simulink model "trirtyfour"  (R2022b)
settings: Solver=VariableStepAuto  StartTime=0.0  StopTime=10.0  RelTol=1e-3
settings Model: Creator=User  LastModifiedBy=User

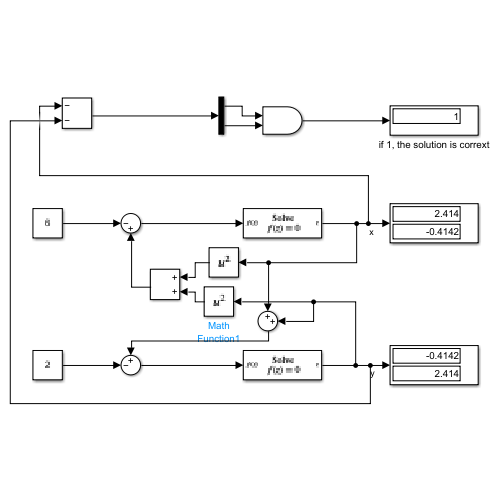
[thumbnail: Simulink's stored preview of the top-level diagram]
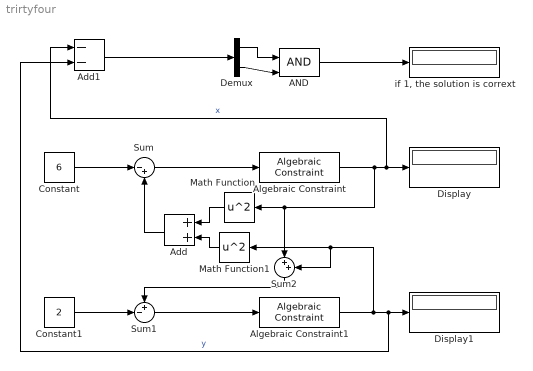
== system trirtyfour ==
  AND : Logic  IconShape=distinctive  AllPortsSameDT=off  OutDataTypeStr=boolean
  Add : Sum
  Add1 : Sum  Inputs=--
  Algebraic Constraint : AlgebraicConstraint  InitialGuess=[1 -1]
  Algebraic Constraint1 : AlgebraicConstraint  InitialGuess=[1 -1]
  Constant : Constant  Value=6
  Constant1 : Constant  Value=2
  Demux : Demux  Outputs=2
  Display : Display
  Display1 : Display
  Math Function : Math  Operator=square
  Math Function1 : Math  Operator=square
  Sum : Sum  Inputs=|-+
  Sum1 : Sum  Inputs=+-|
  Sum2 : Sum  Inputs=|++
  "if 1, the solution is corrext" : Display
  wires:
  Constant/1 -> Sum/1
  Sum/1 -> Algebraic Constraint/1
  Algebraic Constraint/1 -> Sum2/1, Math Function/1, Add1/1, Display/1  "x"
  Add/1 -> Sum/2
  Constant1/1 -> Sum1/2
  Sum1/1 -> Algebraic Constraint1/1
  Algebraic Constraint1/1 -> Sum2/2, Math Function1/1, Add1/2, Display1/1  "y"
  Math Function1/1 -> Add/2
  Math Function/1 -> Add/1
  Sum2/1 -> Sum1/1
  Add1/1 -> Demux/1
  Demux/1 -> AND/1
  Demux/2 -> AND/2
  AND/1 -> "if 1, the solution is corrext"/1
